simulink model "unconnected_lines"  (Simulink 8.2)
settings: Solver=ode45  StartTime=0.0  StopTime=10.0  RelTol=1e-3
settings Model: Creator=ladmin  LastModifiedBy=ladmin
settings DataIOCC: SignalLoggingSaveFormat=Dataset
settings OptimizationCC: ExpressionDepthLimit=128
settings DebuggingCC: FcnCallInpInsideContextMsg=EnableAllAsError  StateNameClashWarn=none
settings GRTTargetCC: CombineOutputUpdateFcns=on  GRTInterface=off

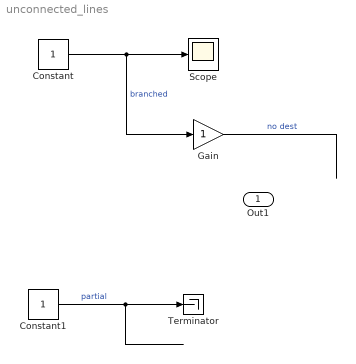
== system unconnected_lines ==
  Constant : Constant
  Constant1 : Constant
  Gain : Gain
  Scope : Scope
  Terminator : Terminator
  Out1 : Outport
  wires:
  Constant/1 -> Gain/1, Scope/1  "branched"
  Gain/1 -> ?  "no dest"
  ? -> Out1/1  "no source"
  ? -> ?  "free"
  Constant1/1 -> Terminator/1  "partial"
